simulink model "sim1el17128"  (R2019b)
settings: Solver=ode45  StartTime=0.0  StopTime=0.5  MaxStep=1e-5  RelTol=1e-3
values from neighbouring files (symbols this model uses):
  ba = Kps    (= 0.627714285714)    [scriptsim1el17128.m]
  Imax = 28    [scriptsim1el17128.m]
  In = 20    [scriptsim1el17128.m]
  J = 0.001    [scriptsim1el17128.m]
  Ki = alphaC*alphaC*L    (= 12067.0225)    [scriptsim1el17128.m]
  Kis = alphaS*Kps    (= 137.908828571)    [scriptsim1el17128.m]
  Kp = alphaC*L    (= 5.4925)    [scriptsim1el17128.m]
  Kps = alphaS*J/psi    (= 0.627714285714)    [scriptsim1el17128.m]
  L = 2.5e-3    (= 0.0025)    [scriptsim1el17128.m]
  psi = 0.35    [scriptsim1el17128.m]
  R = 0.5    [scriptsim1el17128.m]
  Ra = alphaC*L - R    (= 4.9925)    [scriptsim1el17128.m]
  steptime = 0.3    [scriptsim1el17128.m]
  sw1 = 1    [scriptsim1el17128.m]
  sw2 = 1    [scriptsim1el17128.m]
  sw3 = 1    [scriptsim1el17128.m]
  sw4 = 1    [scriptsim1el17128.m]
  tL = tn    (= 7)    [scriptsim1el17128.m]
  Vn = 120    [scriptsim1el17128.m]
  wref = 160    [scriptsim1el17128.m]
settings Model: Creator=Φοιτητικός  LastModifiedBy=user

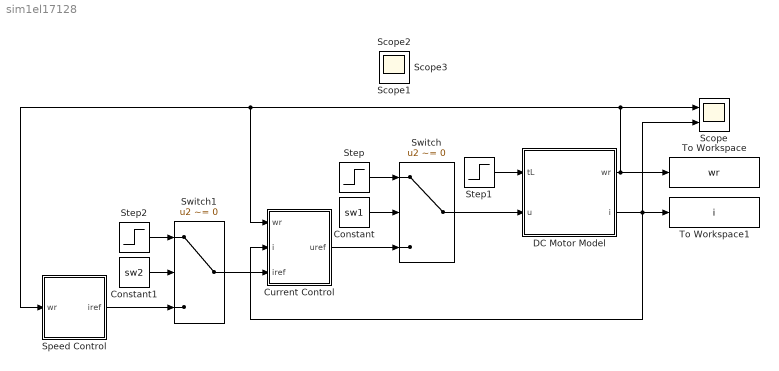
== system sim1el17128 ==
  Constant : Constant  Value=sw1
  Constant1 : Constant  Value=sw2
  Current Control : Subsystem
  DC Motor Model : Subsystem
  Scope : Scope  NumInputPorts=2
  Speed Control : Subsystem
  Step : Step  Time=0.1  After=Vn  SampleTime=0
  Step1 : Step  Time=steptime  After=tL  SampleTime=0
  Step2 : Step  Time=0.1  After=In  SampleTime=0
  Switch : Switch  Criteria=u2 ~= 0  Threshold=1
  Switch1 : Switch  Criteria=u2 ~= 0  Threshold=1
  To Workspace : ToWorkspace  VariableName=wr  SaveFormat=Timeseries  SampleTime=-1
  To Workspace1 : ToWorkspace  VariableName=i  SaveFormat=Timeseries  SampleTime=-1
  Scope1 : Scope
  Scope2 : Scope
  Scope3 : Scope
  wires:
  Step1/1 -> DC Motor Model/1(tL)
  DC Motor Model/1(wr) -> Scope/1, Current Control/1(wr), Speed Control/1(wr), To Workspace/1
  DC Motor Model/2(i) -> Current Control/2(i), To Workspace1/1, Scope/2
  Switch/1 -> DC Motor Model/2(u)
  Step/1 -> Switch/1
  Current Control/1(uref) -> Switch/3
  Constant/1 -> Switch/2
  Constant1/1 -> Switch1/2
  Switch1/1 -> Current Control/3(iref)
  Step2/1 -> Switch1/1
  Speed Control/1(iref) -> Switch1/3

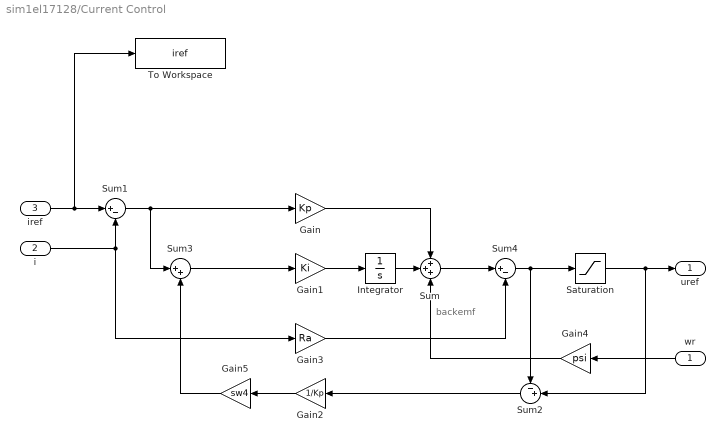
== system sim1el17128/Current Control ==
  note: backemf
  wr : Inport
  i : Inport  Port=2
  iref : Inport  Port=3
  Gain : Gain  Gain=Kp
  Gain1 : Gain  Gain=Ki
  Gain2 : Gain  Gain=1/Kp
  Gain3 : Gain  Gain=Ra
  Gain4 : Gain  Gain=psi
  Gain5 : Gain  Gain=sw4
  Integrator : Integrator
  Saturation : Saturate  UpperLimit=Vn  LowerLimit=-Vn
  Sum : Sum  Inputs=+++
  Sum1 : Sum  Inputs=|+-
  Sum2 : Sum  Inputs=-+|
  Sum3 : Sum  Inputs=|++
  Sum4 : Sum  Inputs=|+-
  To Workspace : ToWorkspace  VariableName=iref  SaveFormat=Timeseries  SampleTime=-1
  uref : Outport
  wires:
  Integrator/1 -> Sum/2
  Gain1/1 -> Integrator/1
  i/1 -> Gain3/1, Sum1/2
  wr/1 -> Gain4/1
  Saturation/1 -> uref/1, Sum2/2
  Gain2/1 -> Gain5/1
  Sum2/1 -> Gain2/1
  Sum3/1 -> Gain1/1
  Sum1/1 -> Gain/1, Sum3/1
  Gain/1 -> Sum/1
  iref/1 -> To Workspace/1, Sum1/1
  Gain4/1 -> Sum/3
  Sum4/1 -> Sum2/1, Saturation/1
  Sum/1 -> Sum4/1
  Gain3/1 -> Sum4/2
  Gain5/1 -> Sum3/2

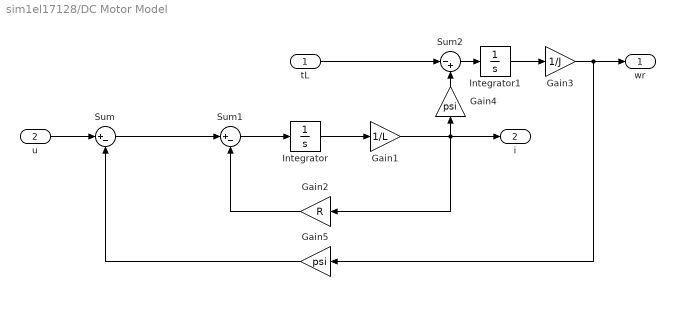
== system sim1el17128/DC Motor Model ==
  tL : Inport
  u : Inport  Port=2
  Gain1 : Gain  Gain=1/L
  Gain2 : Gain  Gain=R
  Gain3 : Gain  Gain=1/J
  Gain4 : Gain  Gain=psi
  Gain5 : Gain  Gain=psi
  Integrator : Integrator
  Integrator1 : Integrator
  Sum : Sum  Inputs=|+-
  Sum1 : Sum  Inputs=|+-
  Sum2 : Sum  Inputs=|-+
  wr : Outport
  i : Outport  Port=2
  wires:
  Gain5/1 -> Sum/2
  Gain4/1 -> Sum2/2
  Gain2/1 -> Sum1/2
  Integrator1/1 -> Gain3/1
  Sum2/1 -> Integrator1/1
  Gain3/1 -> wr/1, Gain5/1
  Integrator/1 -> Gain1/1
  Sum1/1 -> Integrator/1
  Gain1/1 -> Gain2/1, Gain4/1, i/1
  u/1 -> Sum/1
  tL/1 -> Sum2/1
  Sum/1 -> Sum1/1

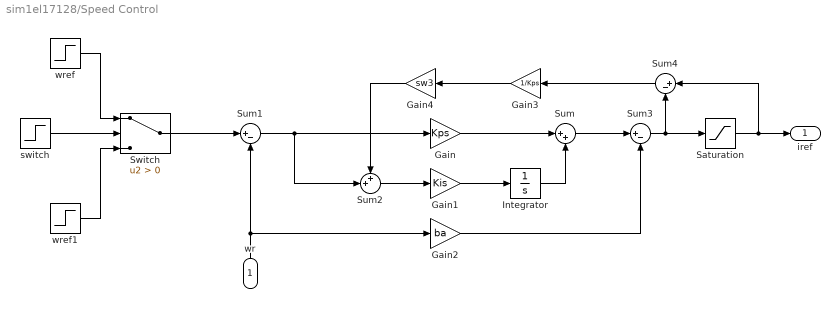
== system sim1el17128/Speed Control ==
  wr : Inport
  Gain : Gain  Gain=Kps
  Gain1 : Gain  Gain=Kis
  Gain2 : Gain  Gain=ba
  Gain3 : Gain  Gain=1/Kps
  Gain4 : Gain  Gain=sw3
  Integrator : Integrator
  Saturation : Saturate  UpperLimit=Imax  LowerLimit=-Imax
  Sum : Sum  Inputs=|++
  Sum1 : Sum  Inputs=|+-
  Sum2 : Sum  Inputs=++|
  Sum3 : Sum  Inputs=|+-
  Sum4 : Sum  Inputs=|+-
  Switch : Switch  Criteria=u2 > Threshold
  switch : Step  Time=0.2  Before=1  After=0  SampleTime=0
  wref : Step  Time=0.1  After=wref  SampleTime=0
  wref1 : Step  Time=0.2  After=314.15  SampleTime=0
  iref : Outport
  wires:
  Sum1/1 -> Sum2/2, Gain/1
  Sum4/1 -> Gain3/1
  Saturation/1 -> iref/1, Sum4/1
  Integrator/1 -> Sum/2
  Sum3/1 -> Saturation/1, Sum4/2
  Sum2/1 -> Gain1/1
  Gain2/1 -> Sum3/2
  Gain1/1 -> Integrator/1
  Gain/1 -> Sum/1
  wr/1 -> Gain2/1, Sum1/2
  Sum/1 -> Sum3/1
  Gain3/1 -> Gain4/1
  Gain4/1 -> Sum2/1
  Switch/1 -> Sum1/1
  wref/1 -> Switch/1
  wref1/1 -> Switch/3
  switch/1 -> Switch/2
